simulink model "Synchr_Gen5"  (Simulink 4.00)
settings: Solver=ode23tb  StartTime=0.0  StopTime=5  RelTol=1e-3
InitFcn:
  | powericon('psbinitsys',bdroot);
libraries: powerlib2 x7, powerlib11 x1
settings Model: LastModifiedBy=ieao

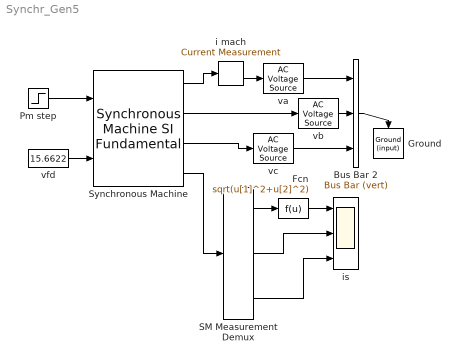
== system Synchr_Gen5 ==
  Bus Bar 2 : powerlib2/Connectors/Bus Bar (vert)  Tag=PoWeRsYsTeMbLoCk  entrees=3  sorties=1  PSBOutputType=11111111111111111111111111111111111111111111111111111111111111111111111111111111111111111
  Fcn : Fcn  Expr=sqrt(u[1]^2+u[2]^2)
  Ground : powerlib2/Connectors/Ground (input)  Tag=PoWeRsYsTeMbLoCk  Orientation=down
  Pm step : Step  Time=2  Before=-50000  After=-60000  SampleTime=0
  SM Measurement Demux : powerlib11/Machines/SM Measurement Demux  a=off  b=on  c=off  d=off  e=off  f=off  g=off  h=on  i=on  j=off
  Synchronous Machine : powerlib2/Machines/Synchronous Machine SI Fundamental  Tag=PoWeRsYsTeMbLoCk  rotorType=Salient-pole  x1="[ 111900 440*sqrt(3) 50  0]"  x2=[ .26 1.14e-3 13.7e-3 11.0e-3 ]  x3=[ 0.13 2.1e-3 ]  x4b=[ 1 2 3 4 5 6 ]  x4=[ 0.0224 1.4e-3 0.02 1e-3 ]  x5=[ 24.9 0 2 ]  x6="[ 0  335.978  55.9962,55.9962,55.9962  258.5352,138.5352,18.5352  15.6622 ]"  x7=off  x8=[]  x9=off  PSBOutputType=1110  iounits=1
  i mach : powerlib2/Measurements/Current Measurement  Tag=PoWeRsYsTeMmEaSuReMeNt  PSBOutputType=01  PSBequivalent=1
  is : Scope  NumInputPorts=3
      settings: TimeRange=auto  YMin=55~-5~-5  YMax=75~5~5  SaveToWorkspace=off  SaveName=is  DataFormat=Array  MaxDataPoints=5000
  va : powerlib2/Electrical Sources/AC Voltage Source  Tag=PoWeRsYsTeMbLoCk  A=440*sqrt(2)  P=270  F=50  stime=0  mesure=None  PSBOutputType=1
  vb : powerlib2/Electrical Sources/AC Voltage Source  Tag=PoWeRsYsTeMbLoCk  A=440*sqrt(2)  P=150  F=50  stime=0  mesure=None  PSBOutputType=1
  vc : powerlib2/Electrical Sources/AC Voltage Source  Tag=PoWeRsYsTeMbLoCk  A=440*sqrt(2)  P=30  F=50  stime=0  mesure=None  PSBOutputType=1
  vfd : Constant  Value=15.6622
  wires:
  Synchronous Machine/4 -> SM Measurement Demux/1
  vfd/1 -> Synchronous Machine/2
  Synchronous Machine/2 -> vb/1
  va/1 -> Bus Bar 2/1
  vb/1 -> Bus Bar 2/2
  vc/1 -> Bus Bar 2/3
  Bus Bar 2/1 -> Ground/1
  i mach/2 -> va/1
  Synchronous Machine/1 -> i mach/1
  Pm step/1 -> Synchronous Machine/1
  Fcn/1 -> is/1
  SM Measurement Demux/1 -> Fcn/1
  SM Measurement Demux/2 -> is/2
  SM Measurement Demux/3 -> is/3
  Synchronous Machine/3 -> vc/1
